simulink model "HR_Stateflow_Control"  (R2020b)
settings: Solver=VariableStepAuto  StartTime=0.0  StopTime=inf  MaxStep=1E-4  RelTol=1e-9
undefined symbols (not defined in the file): Dgain, g, Igain, initHeight, L1, L2, M, m1, m2, massTot, Pgain, physParam, tau1, tau2, th1o, th2o, yCMo
libraries: pid_lib x2, simulink x2
settings Model: Creator=Bradley Kwan  LastModifiedBy=Bradley Kwan
settings DebuggingCC: AlgebraicLoopMsg=none

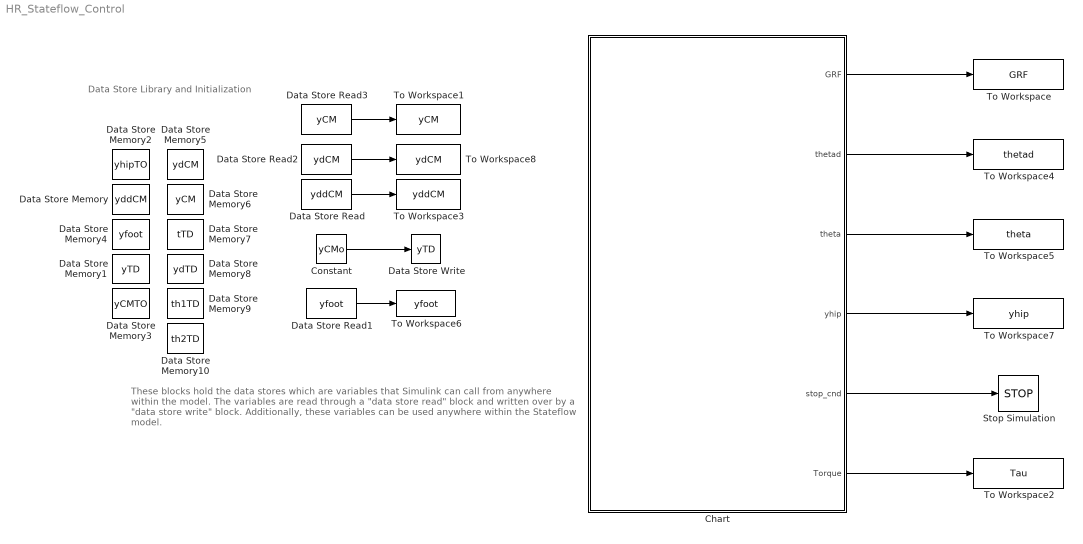
== system HR_Stateflow_Control ==
  note: These blocks hold the data stores which are variables that Simulink can call from anywhere within the model. The variables are read through a "data store read" block and written over by a "data store write" block. Additionally, these variables can be used anywhere within the Stateflow model.
  note: Data Store Library and Initialization
  Chart : Stateflow chart  TreatAsAtomicUnit=on
  Constant : Constant  Value=yCMo
  Data Store Memory : DataStoreMemory  DataStoreName=yddCM  ShowAdditionalParam=off  OutDataTypeStr=double
      settings: LockScale=on
  Data Store Memory1 : DataStoreMemory  DataStoreName=yTD  ShowAdditionalParam=off  OutDataTypeStr=double
      settings: LockScale=on
  Data Store Memory10 : DataStoreMemory  DataStoreName=th2TD  ShowAdditionalParam=off  OutDataTypeStr=double
      settings: LockScale=on
  Data Store Memory2 : DataStoreMemory  DataStoreName=yhipTO  ShowAdditionalParam=off  OutDataTypeStr=double
      settings: LockScale=on
  Data Store Memory3 : DataStoreMemory  DataStoreName=yCMTO  ShowAdditionalParam=off  OutDataTypeStr=double
      settings: LockScale=on
  Data Store Memory4 : DataStoreMemory  DataStoreName=yfoot  ShowAdditionalParam=off  OutDataTypeStr=double
      settings: LockScale=on
  Data Store Memory5 : DataStoreMemory  DataStoreName=ydCM  ShowAdditionalParam=off  OutDataTypeStr=double
      settings: LockScale=on
  Data Store Memory6 : DataStoreMemory  DataStoreName=yCM  ShowAdditionalParam=off  OutDataTypeStr=double
      settings: LockScale=on
  Data Store Memory7 : DataStoreMemory  DataStoreName=tTD  ShowAdditionalParam=off  OutDataTypeStr=double
      settings: LockScale=on
  Data Store Memory8 : DataStoreMemory  DataStoreName=ydTD  ShowAdditionalParam=off  OutDataTypeStr=double
      settings: LockScale=on
  Data Store Memory9 : DataStoreMemory  DataStoreName=th1TD  ShowAdditionalParam=off  OutDataTypeStr=double
      settings: LockScale=on
  Data Store Read : DataStoreRead  DataStoreName=yddCM
  Data Store Read1 : DataStoreRead  DataStoreName=yfoot
  Data Store Read2 : DataStoreRead  DataStoreName=ydCM
  Data Store Read3 : DataStoreRead  DataStoreName=yCM
  Data Store Write : DataStoreWrite  DataStoreName=yTD
  Stop Simulation : Stop
  To Workspace : ToWorkspace  VariableName=GRF  SampleTime=-1
  To Workspace1 : ToWorkspace  VariableName=yCM  SampleTime=-1
  To Workspace2 : ToWorkspace  VariableName=Tau  SampleTime=-1
  To Workspace3 : ToWorkspace  VariableName=yddCM  SampleTime=-1
  To Workspace4 : ToWorkspace  VariableName=thetad  SampleTime=-1
  To Workspace5 : ToWorkspace  VariableName=theta  SampleTime=-1
  To Workspace6 : ToWorkspace  VariableName=yfoot  SampleTime=-1
  To Workspace7 : ToWorkspace  VariableName=yhip  SampleTime=-1
  To Workspace8 : ToWorkspace  VariableName=ydCM  SampleTime=-1
  wires:
  Chart/1(GRF) -> To Workspace/1
  Chart/5(stop_cnd) -> Stop Simulation/1
  Data Store Read/1 -> To Workspace3/1
  Chart/2(thetad) -> To Workspace4/1
  Chart/3(theta) -> To Workspace5/1
  Constant/1 -> Data Store Write/1
  Chart/4(yhip) -> To Workspace7/1
  Data Store Read1/1 -> To Workspace6/1
  Data Store Read2/1 -> To Workspace8/1
  Data Store Read3/1 -> To Workspace1/1
  Chart/6(Torque) -> To Workspace2/1

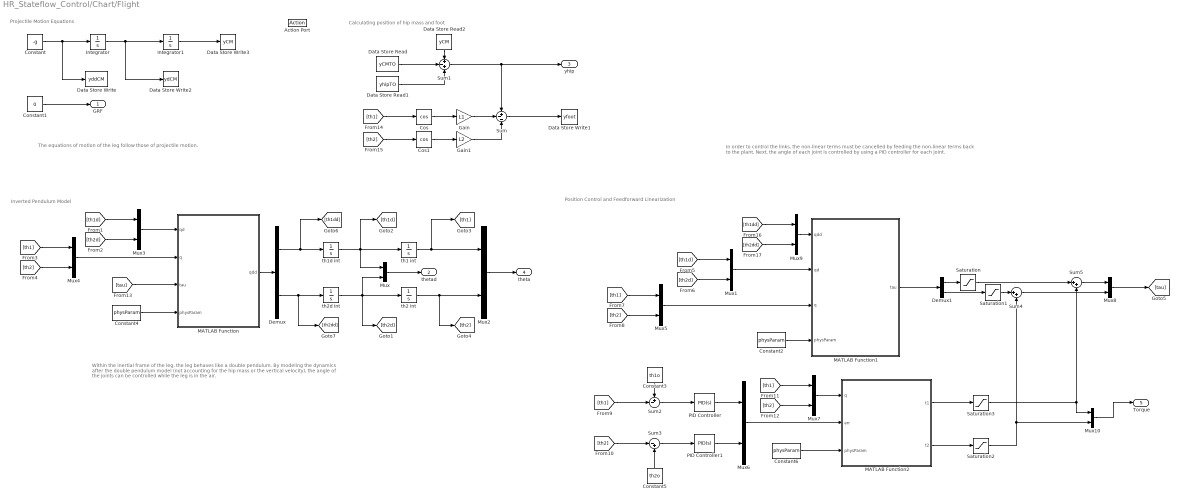
== system HR_Stateflow_Control/Chart/Flight ==
  note: The equations of motion of the leg follow those of projectile motion.
  note: In order to control the links, the non-linear terms must be cancelled by feeding the non-linear terms back to the plant. Next, the angle of each joint is controlled by using a PID controller for each joint.
  note: Within the inertial frame of the leg, the leg behaves like a double pendulum. By modeling the dynamics after the double pendulum model (not accounting for the hip mass or the vertical velocity), the angle of the joints can be controlled while the leg is in the air.
  note: Position Control and Feedforward Linearization
  note: Inverted Pendulum Model
  note: Calculating position of hip mass and foot
  note: Projectile Motion Equations
  Action Port : ActionPort
      settings: CopyFcn=Stateflow.SLINSF.SimulinkMan.removeBlockPreDeleteFcn  PreDeleteFcn=Stateflow.SLINSF.SimulinkMan.unsafePredeleteFcn
  Constant : Constant  Value=-g
  Constant1 : Constant  Value=0
  Constant2 : Constant  Value=physParam
  Constant3 : Constant  Value=th1o
  Constant4 : Constant  Value=physParam
  Constant5 : Constant  Value=th2o
  Constant6 : Constant  Value=physParam
  Cos : Trigonometry  Operator=cos
  Cos1 : Trigonometry  Operator=cos
  Data Store Read : DataStoreRead  DataStoreName=yCMTO
  Data Store Read1 : DataStoreRead  DataStoreName=yhipTO
  Data Store Read2 : DataStoreRead  DataStoreName=yCM
  Data Store Write : DataStoreWrite  DataStoreName=yddCM
  Data Store Write1 : DataStoreWrite  DataStoreName=yfoot
  Data Store Write2 : DataStoreWrite  DataStoreName=ydCM
  Data Store Write3 : DataStoreWrite  DataStoreName=yCM
  Demux : Demux  Outputs=2
  Demux1 : Demux  Outputs=2
  Gain : Gain  Gain=L1
  Gain1 : Gain  Gain=L2
  Integrator : Integrator  ContinuousStateAttributes='ydCM'
  Integrator1 : Integrator  InitialCondition=initHeight  ContinuousStateAttributes='yCM'
  MATLAB Function : MATLAB Function  TreatAsAtomicUnit=on
  MATLAB Function1 : MATLAB Function  TreatAsAtomicUnit=on
  MATLAB Function2 : MATLAB Function  TreatAsAtomicUnit=on
  Mux{,1..10} (11 alike) : Mux  Inputs=2
  PID Controller : pid_lib/PID Controller  Controller=PID  Form=Parallel  TimeDomain=Continuous-time  UseExternalTs=off  SampleTime=-1  IntegratorMethod=Forward Euler  FilterMethod=Forward Euler  ControllerParametersSource=internal  P=Pgain  I=Igain  D=Dgain  UseFilter=on  N=100  TunerSelectOption=Transfer Function Based (PID Tuner App)  InitialConditionSource=internal  InitialConditionForIntegrator=0  InitialConditionForFilter=0  DifferentiatorICPrevScaledInput=0  ExternalReset=none  TrackingMode=off  Kt=1  LimitOutput=off  SatLimitsSource=internal  UpperSaturationLimit=inf  LowerSaturationLimit=-inf  LinearizeAsGain=on  AntiWindupMode=none  Kb=1  POutMin=[]  POutMax=[]  IOutMin=[]  IOutMax=[]  DOutMin=[]  DOutMax=[]  NOutMin=[]  NOutMax=[]  SumOutMin=[]  SumOutMax=[]  SaturationOutMin=[]  SaturationOutMax=[]  PParamMin=[]  PParamMax=[]  IParamMin=[]  IParamMax=[]  DParamMin=[]  DParamMax=[]  NParamMin=[]  NParamMax=[]  KbParamMin=[]  KbParamMax=[]  KtParamMin=[]  KtParamMax=[]  KbOutMin=[]  KbOutMax=[]  KtOutMin=[]  KtOutMax=[]  IntegratorOutMin=[]  IntegratorOutMax=[]  FilterOutMin=[]  FilterOutMax=[]  SumI1OutMin=[]  SumI1OutMax=[]  SumI2OutMin=[]  SumI2OutMax=[]  SumI3OutMin=[]  SumI3OutMax=[]  SumI4OutMin=[]  SumI4OutMax=[]  SumDOutMin=[]  SumDOutMax=[]  DifferentiatorOutMin=[]  DifferentiatorOutMax=[]  FilterDiffOutCoefMin=[]  FilterDiffOutCoefMax=[]  ReciprocalOutMin=[]  ReciprocalOutMax=[]  SumDenOutMin=[]  SumDenOutMax=[]  SumNumOutMin=[]  SumNumOutMax=[]  DivideOutMin=[]  DivideOutMax=[]  UdiffTsProdOutMin=[]  UdiffTsProdOutMax=[]  NTsProdOutMin=[]  NTsProdOutMax=[]  UintegralTsProdOutMin=[]  UintegralTsProdOutMax=[]  UngainTsProdOutMin=[]  UngainTsProdOutMax=[]  IntegratorContinuousStateAttributes=''  IntegratorStateMustResolveToSignalObject=off  IntegratorRTWStateStorageClass=Auto  FilterContinuousStateAttributes=''  FilterStateMustResolveToSignalObject=off  FilterRTWStateStorageClass=Auto  ParallelPVariant=InternalParameters  IdealPVariant=Disabled  IVariant=InternalParameters  DVariant=InternalParameters  IntegratorVariant=Continuous  SatVariant=Disabled  AWVariant=Passthrough  PCopyVariant=Disabled  TRVariant=Disabled  FdbkBlocksVariant=Forward  IdealPFdbkVariant=Disabled  SatFdbkVariant=Disabled  DerivativeFilterVariant=ContFilter  NVariant=InternalParameters  NCopyVariant=Disabled  FilterICVariant=InternalICsFilter  IntegratorICVariant=InternalICs  ExternalResetVariant=Disabled  TRSumVariant=Passthrough  SumFdbkVariant=Disabled  SumVariant=Sum_PID  TsampFilterVariant=InternalTs  TsampNgainVariant=Passthrough  TsampIntegralVariant=Passthrough  ExternalSaturationOutDataTypeStr=Inherit: Same as second input
  PID Controller1 : pid_lib/PID Controller  Controller=PID  Form=Parallel  TimeDomain=Continuous-time  UseExternalTs=off  SampleTime=-1  IntegratorMethod=Forward Euler  FilterMethod=Forward Euler  ControllerParametersSource=internal  P=Pgain  I=Igain  D=Dgain  UseFilter=on  N=100  TunerSelectOption=Transfer Function Based (PID Tuner App)  InitialConditionSource=internal  InitialConditionForIntegrator=0  InitialConditionForFilter=0  DifferentiatorICPrevScaledInput=0  ExternalReset=none  TrackingMode=off  Kt=1  LimitOutput=off  SatLimitsSource=internal  UpperSaturationLimit=inf  LowerSaturationLimit=-inf  LinearizeAsGain=on  AntiWindupMode=none  Kb=1  POutMin=[]  POutMax=[]  IOutMin=[]  IOutMax=[]  DOutMin=[]  DOutMax=[]  NOutMin=[]  NOutMax=[]  SumOutMin=[]  SumOutMax=[]  SaturationOutMin=[]  SaturationOutMax=[]  PParamMin=[]  PParamMax=[]  IParamMin=[]  IParamMax=[]  DParamMin=[]  DParamMax=[]  NParamMin=[]  NParamMax=[]  KbParamMin=[]  KbParamMax=[]  KtParamMin=[]  KtParamMax=[]  KbOutMin=[]  KbOutMax=[]  KtOutMin=[]  KtOutMax=[]  IntegratorOutMin=[]  IntegratorOutMax=[]  FilterOutMin=[]  FilterOutMax=[]  SumI1OutMin=[]  SumI1OutMax=[]  SumI2OutMin=[]  SumI2OutMax=[]  SumI3OutMin=[]  SumI3OutMax=[]  SumI4OutMin=[]  SumI4OutMax=[]  SumDOutMin=[]  SumDOutMax=[]  DifferentiatorOutMin=[]  DifferentiatorOutMax=[]  FilterDiffOutCoefMin=[]  FilterDiffOutCoefMax=[]  ReciprocalOutMin=[]  ReciprocalOutMax=[]  SumDenOutMin=[]  SumDenOutMax=[]  SumNumOutMin=[]  SumNumOutMax=[]  DivideOutMin=[]  DivideOutMax=[]  UdiffTsProdOutMin=[]  UdiffTsProdOutMax=[]  NTsProdOutMin=[]  NTsProdOutMax=[]  UintegralTsProdOutMin=[]  UintegralTsProdOutMax=[]  UngainTsProdOutMin=[]  UngainTsProdOutMax=[]  IntegratorContinuousStateAttributes=''  IntegratorStateMustResolveToSignalObject=off  IntegratorRTWStateStorageClass=Auto  FilterContinuousStateAttributes=''  FilterStateMustResolveToSignalObject=off  FilterRTWStateStorageClass=Auto  ParallelPVariant=InternalParameters  IdealPVariant=Disabled  IVariant=InternalParameters  DVariant=InternalParameters  IntegratorVariant=Continuous  SatVariant=Disabled  AWVariant=Passthrough  PCopyVariant=Disabled  TRVariant=Disabled  FdbkBlocksVariant=Forward  IdealPFdbkVariant=Disabled  SatFdbkVariant=Disabled  DerivativeFilterVariant=ContFilter  NVariant=InternalParameters  NCopyVariant=Disabled  FilterICVariant=InternalICsFilter  IntegratorICVariant=InternalICs  ExternalResetVariant=Disabled  TRSumVariant=Passthrough  SumFdbkVariant=Disabled  SumVariant=Sum_PID  TsampFilterVariant=InternalTs  TsampNgainVariant=Passthrough  TsampIntegralVariant=Passthrough  ExternalSaturationOutDataTypeStr=Inherit: Same as second input
  Saturation : Saturate  UpperLimit=8  LowerLimit=-8
  Saturation1 : Saturate  UpperLimit=8  LowerLimit=-8
  Saturation2 : Saturate  UpperLimit=5  LowerLimit=-5
  Saturation3 : Saturate  UpperLimit=5  LowerLimit=-5
  Sum : Sum  Inputs=+--
  Sum1 : Sum  Inputs=+-+
  Sum2 : Sum  Inputs=+-|
  Sum3 : Sum  Inputs=|-+
  Sum4 : Sum  Inputs=|++
  Sum5 : Sum  Inputs=|++
  th1 int : Integrator  InitialCondition=th1o  ContinuousStateAttributes='th1'
  th1d int : Integrator  ContinuousStateAttributes='th1d'
  th2 int : Integrator  InitialCondition=th2o  ContinuousStateAttributes='th2'
  th2d int : Integrator  ContinuousStateAttributes='th2d'
  GRF : Outport
  thetad : Outport  Port=2
  yhip : Outport  Port=3
  theta : Outport  Port=4
  Torque : Outport  Port=5
  wires:
  Constant1/1 -> GRF/1
  Constant/1 -> Data Store Write/1, Integrator/1
  Integrator/1 -> Data Store Write2/1, Integrator1/1
  Integrator1/1 -> Data Store Write3/1
  Cos/1 -> Gain/1
  Cos1/1 -> Gain1/1
  Gain/1 -> Sum/2
  Gain1/1 -> Sum/3
  Sum/1 -> Data Store Write1/1
  Data Store Read/1 -> Sum1/2
  Data Store Read2/1 -> Sum1/1
  Data Store Read1/1 -> Sum1/3
  Sum1/1 -> Sum/1, yhip/1
  MATLAB Function/1(qdd) -> Demux/1
  th1d int/1 -> Mux/1, th1 int/1, [th1d]
  th2d int/1 -> Mux/2, [th2d], th2 int/1
  th1 int/1 -> [th1], Mux2/1
  th2 int/1 -> [th2], Mux2/2
  Constant4/1 -> MATLAB Function/4(physParam)
  [th1d] -> Mux3/1
  [th2d] -> Mux3/2
  Mux3/1 -> MATLAB Function/1(qd)
  [th2] -> Mux4/2
  [th1] -> Mux4/1
  Mux4/1 -> MATLAB Function/2(q)
  Constant2/1 -> MATLAB Function1/4(physParam)
  Mux5/1 -> MATLAB Function1/3(q)
  [th1] -> Mux5/1
  [th2] -> Mux5/2
  Mux1/1 -> MATLAB Function1/2(qd)
  [th2d] -> Mux1/2
  [th1d] -> Mux1/1
  MATLAB Function1/1(tau) -> Demux1/1
  [th2] -> Sum3/1
  [th1] -> Sum2/2
  Constant3/1 -> Sum2/1
  Constant5/1 -> Sum3/2
  Sum2/1 -> PID Controller/1
  Sum3/1 -> PID Controller1/1
  PID Controller/1 -> Mux6/1
  PID Controller1/1 -> Mux6/2
  Mux6/1 -> MATLAB Function2/2(err)
  [th2] -> Mux7/2
  [th1] -> Mux7/1
  Mux7/1 -> MATLAB Function2/1(q)
  Constant6/1 -> MATLAB Function2/3(physParam)
  Mux2/1 -> theta/1
  MATLAB Function2/1(t1) -> Saturation3/1
  Sum5/1 -> Mux8/1
  Sum4/1 -> Mux8/2
  Mux8/1 -> [tau]
  [tau] -> MATLAB Function/3(tau)
  Demux/1 -> [th1dd], th1d int/1
  Demux/2 -> [th2dd], th2d int/1
  [th1] -> Cos/1
  [th2] -> Cos1/1
  Mux/1 -> thetad/1
  Demux1/1 -> Saturation/1
  Saturation/1 -> Sum5/1
  Demux1/2 -> Saturation1/1
  Saturation1/1 -> Sum4/1
  [th1dd] -> Mux9/1
  [th2dd] -> Mux9/2
  Mux9/1 -> MATLAB Function1/1(qdd)
  Mux10/1 -> Torque/1
  MATLAB Function2/2(t2) -> Saturation2/1
  Saturation3/1 -> Sum5/2, Mux10/1
  Saturation2/1 -> Sum4/2, Mux10/2

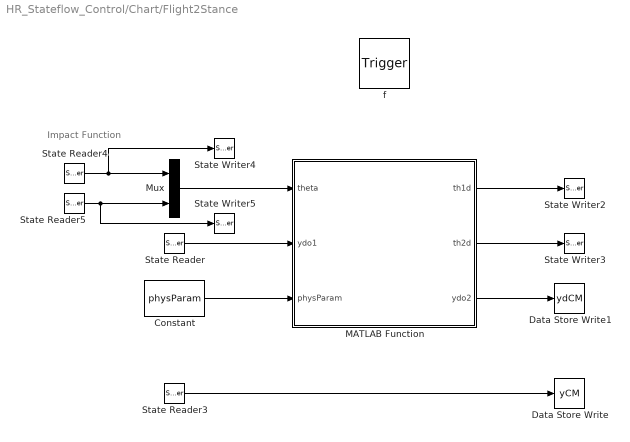
== system HR_Stateflow_Control/Chart/Flight2Stance ==
  note: Impact Function
  f : TriggerPort  TriggerType=function-call  VariantControl=(inherit)
      settings: CopyFcn=Stateflow.SLINSF.SimulinkMan.removeBlockPreDeleteFcn  PreDeleteFcn=Stateflow.SLINSF.SimulinkMan.unsafePredeleteFcn
  Constant : Constant  Value=physParam
  Data Store Write : DataStoreWrite  DataStoreName=yCM
  Data Store Write1 : DataStoreWrite  DataStoreName=ydCM
  MATLAB Function : MATLAB Function  TreatAsAtomicUnit=on
  Mux : Mux  Inputs=2
  State Reader : StateReader  StateOwnerBlock=../../Flight/Integrator  StateName=ydCM
  State Reader3 : StateReader  StateOwnerBlock=../../Flight/Integrator1  StateName=yCM
  State Reader4 : StateReader  StateOwnerBlock=../../Flight/th1 int  StateName=th1
  State Reader5 : StateReader  StateOwnerBlock=../../Flight/th2 int  StateName=th2
  State Writer2 : StateWriter  StateOwnerBlock=../../Stance/th1d int.  StateName=th1d
  State Writer3 : StateWriter  StateOwnerBlock=../../Stance/th2d int.  StateName=th2d
  State Writer4 : StateWriter  StateOwnerBlock=../../Stance/th1 int.  StateName=th1
  State Writer5 : StateWriter  StateOwnerBlock=../../Stance/th2 int.  StateName=th2
  wires:
  State Reader/1 -> MATLAB Function/2(ydo1)
  State Reader4/1 -> Mux/1, State Writer4/1
  Mux/1 -> MATLAB Function/1(theta)
  Constant/1 -> MATLAB Function/3(physParam)
  MATLAB Function/3(ydo2) -> Data Store Write1/1
  State Reader3/1 -> Data Store Write/1
  MATLAB Function/1(th1d) -> State Writer2/1
  MATLAB Function/2(th2d) -> State Writer3/1
  State Reader5/1 -> Mux/2, State Writer5/1

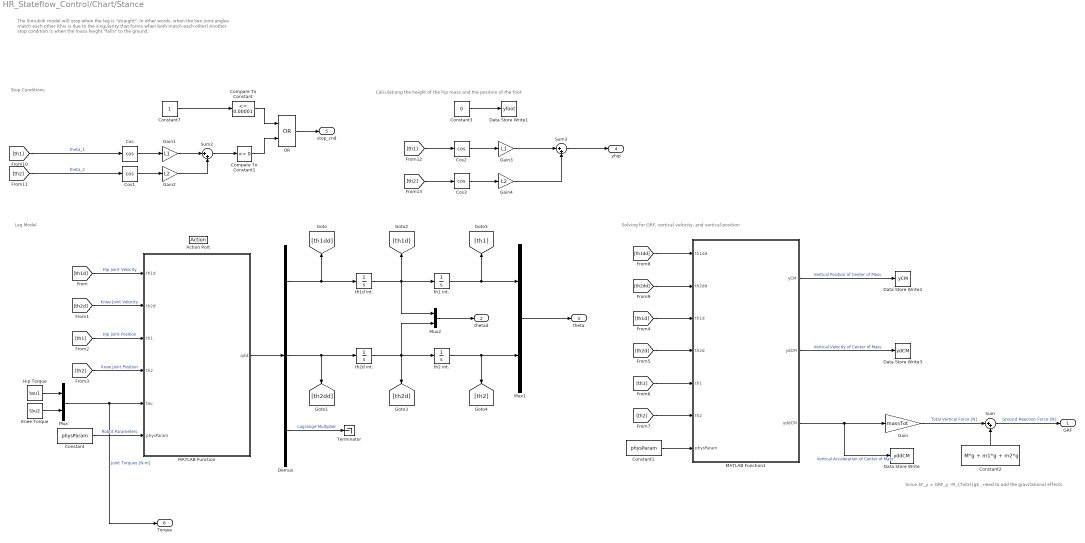
== system HR_Stateflow_Control/Chart/Stance ==
  note: Calculatiung the height of the hip mass and the position of the foot
  note: Solving for GRF, vertical velocity, and vertical position
  note: Leg Model
  note: Since $F_y = GRF_y -M_{Total}g$ , need to add the gravitational effects
  note: Stop Conditions
  note: The Simulink model will stop when the leg is "straight". In other words, when the two joint angles match each other (this is due to the singularity that forms when both match each other)
      |
      | Another stop condition is when the mass height "falls" to the ground.
  Action Port : ActionPort
      settings: CopyFcn=Stateflow.SLINSF.SimulinkMan.removeBlockPreDeleteFcn  PreDeleteFcn=Stateflow.SLINSF.SimulinkMan.unsafePredeleteFcn
  Compare To Constant : simulink/Logic and Bit Operations/Compare To Constant  relop=<=  const=0.00001  OutDataTypeStr=boolean
  Compare To Constant1 : simulink/Logic and Bit Operations/Compare To Constant  relop=<=  const=0  OutDataTypeStr=boolean
  Constant : Constant  Value=physParam
  Constant1 : Constant  Value=physParam
  Constant2 : Constant  Value=M*g + m1*g + m2*g
  Constant3 : Constant  Value=0
  Constant7 : Constant
  Cos{,1..3} (4 alike) : Trigonometry  Operator=cos
  Data Store Write : DataStoreWrite  DataStoreName=yddCM
  Data Store Write1 : DataStoreWrite  DataStoreName=yfoot
  Data Store Write2 : DataStoreWrite  DataStoreName=yCM
  Data Store Write3 : DataStoreWrite  DataStoreName=ydCM
  Demux : Demux  Outputs=3
  Gain : Gain  Gain=massTot
  Gain1 : Gain  Gain=L1
  Gain2 : Gain  Gain=L2
  Gain3 : Gain  Gain=L1
  Gain4 : Gain  Gain=L2
  Hip Torque : Constant  Value=tau1
  Knee Torque : Constant  Value=tau2
  MATLAB Function : MATLAB Function  TreatAsAtomicUnit=on
  MATLAB Function1 : MATLAB Function  TreatAsAtomicUnit=on
  Mux : Mux  Inputs=2
  Mux1 : Mux  Inputs=2
  Mux2 : Mux  Inputs=2
  OR : Logic  Operator=OR  IconShape=distinctive  AllPortsSameDT=off  OutDataTypeStr=boolean
  Sum : Sum  Inputs=|++
  Sum2 : Sum  Inputs=|++
  Sum3 : Sum  Inputs=|++
  Terminator : Terminator
  th1 int. : Integrator  InitialCondition=th1o  ContinuousStateAttributes='th1'
  th1d int. : Integrator  ContinuousStateAttributes='th1d'
  th2 int. : Integrator  InitialCondition=th2o  ContinuousStateAttributes='th2'
  th2d int. : Integrator  ContinuousStateAttributes='th2d'
  GRF : Outport
  thetad : Outport  Port=2
  theta : Outport  Port=3
  yhip : Outport  Port=4
  stop_cnd : Outport  Port=5
  Torque : Outport  Port=6
  wires:
  Knee Torque/1 -> Mux/2
  Hip Torque/1 -> Mux/1
  Mux/1 -> Torque/1, MATLAB Function/5(tau)  "Joint Torques [N-m]"
  Constant/1 -> MATLAB Function/6(physParam)  "Robot Parameters"
  [th1d] -> MATLAB Function/1(th1d)  "Hip Joint Velocity"
  [th2d] -> MATLAB Function/2(th2d)  "Knee Joint Velocity"
  [th1] -> MATLAB Function/3(th1)  "Hip Joint Position"
  [th2] -> MATLAB Function/4(th2)  "Knee Joint Position"
  MATLAB Function/1(qdd) -> Demux/1
  Demux/1 -> [th1dd], th1d int./1
  Demux/2 -> [th2dd], th2d int./1
  th1d int./1 -> Mux2/1, th1 int./1, [th1d]
  th2d int./1 -> Mux2/2, [th2d], th2 int./1
  Mux1/1 -> theta/1
  th1 int./1 -> [th1], Mux1/1
  th2 int./1 -> [th2], Mux1/2
  Demux/3 -> Terminator/1  "Lagrange Multiplier"
  Mux2/1 -> thetad/1
  Constant1/1 -> MATLAB Function1/7(physParam)
  [th2] -> MATLAB Function1/6(th2)
  [th1] -> MATLAB Function1/5(th1)
  [th2d] -> MATLAB Function1/4(th2d)
  [th1d] -> MATLAB Function1/3(th1d)
  [th2dd] -> MATLAB Function1/2(th2dd)
  [th1dd] -> MATLAB Function1/1(th1dd)
  MATLAB Function1/3(yddCM) -> Data Store Write/1, Gain/1  "Vertical Acceleration of Center of Mass"
  Gain/1 -> Sum/1  "Total Vertical Force [N]"
  Constant2/1 -> Sum/2
  Gain2/1 -> Sum2/2
  OR/1 -> stop_cnd/1
  Compare To Constant/1 -> OR/1
  Cos1/1 -> Gain2/1
  [th1] -> Cos/1  "theta_1"
  [th2] -> Cos1/1  "theta_2"
  Sum2/1 -> Compare To Constant1/1
  Cos/1 -> Gain1/1
  Compare To Constant1/1 -> OR/2
  Gain1/1 -> Sum2/1
  Sum/1 -> GRF/1  "Ground Reaction Force [N]"
  Constant3/1 -> Data Store Write1/1
  [th1] -> Cos2/1
  [th2] -> Cos3/1
  Cos2/1 -> Gain3/1
  Cos3/1 -> Gain4/1
  Gain3/1 -> Sum3/1
  Gain4/1 -> Sum3/2
  Sum3/1 -> yhip/1
  MATLAB Function1/1(yCM) -> Data Store Write2/1  "Vertical Position of Center of Mass"
  MATLAB Function1/2(ydCM) -> Data Store Write3/1  "Vertical Velocity of Center of Mass"
  Constant7/1 -> Compare To Constant/1

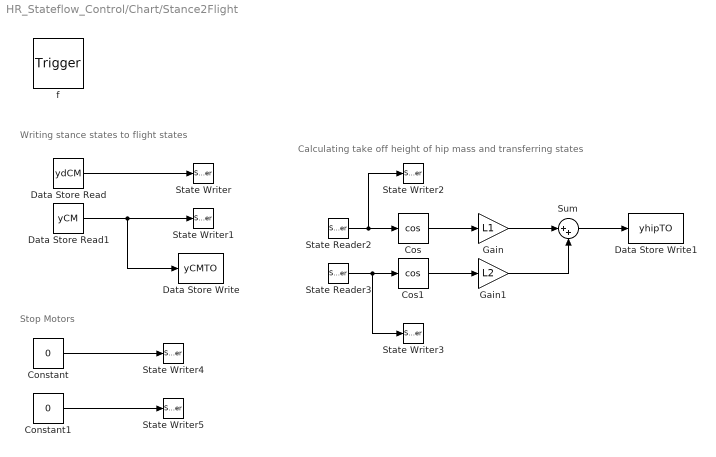
== system HR_Stateflow_Control/Chart/Stance2Flight ==
  note: Calculating take off height of hip mass and transferring states
  note: Writing stance states to flight states
  note: Stop Motors
  f : TriggerPort  TriggerType=function-call  VariantControl=(inherit)
      settings: CopyFcn=Stateflow.SLINSF.SimulinkMan.removeBlockPreDeleteFcn  PreDeleteFcn=Stateflow.SLINSF.SimulinkMan.unsafePredeleteFcn
  Constant : Constant  Value=0
  Constant1 : Constant  Value=0
  Cos : Trigonometry  Operator=cos
  Cos1 : Trigonometry  Operator=cos
  Data Store Read : DataStoreRead  DataStoreName=ydCM
  Data Store Read1 : DataStoreRead  DataStoreName=yCM
  Data Store Write : DataStoreWrite  DataStoreName=yCMTO
  Data Store Write1 : DataStoreWrite  DataStoreName=yhipTO
  Gain : Gain  Gain=L1
  Gain1 : Gain  Gain=L2
  State Reader2 : StateReader  StateOwnerBlock=../../Stance/th1 int.  StateName=th1
  State Reader3 : StateReader  StateOwnerBlock=../../Stance/th2 int.  StateName=th2
  State Writer : StateWriter  StateOwnerBlock=../../Flight/Integrator  StateName=ydCM
  State Writer1 : StateWriter  StateOwnerBlock=../../Flight/Integrator1  StateName=yCM
  State Writer2 : StateWriter  StateOwnerBlock=../../Flight/th1 int  StateName=th1
  State Writer3 : StateWriter  StateOwnerBlock=../../Flight/th2 int  StateName=th2
  State Writer4 : StateWriter  StateOwnerBlock=../../Flight/th1d int  StateName=th1d
  State Writer5 : StateWriter  StateOwnerBlock=../../Flight/th2d int  StateName=th2d
  Sum : Sum  Inputs=|++
  wires:
  Data Store Read/1 -> State Writer/1
  Gain1/1 -> Sum/2
  Gain/1 -> Sum/1
  Cos1/1 -> Gain1/1
  State Reader2/1 -> State Writer2/1, Cos/1
  Sum/1 -> Data Store Write1/1
  Cos/1 -> Gain/1
  Data Store Read1/1 -> Data Store Write/1, State Writer1/1
  State Reader3/1 -> State Writer3/1, Cos1/1
  Constant/1 -> State Writer4/1
  Constant1/1 -> State Writer5/1

== matlab function HR_Stateflow_Control/Chart/Flight2Stance/MATLAB Function ==
  data: theta input; th1d output; ydo1 input; physParam input; th2d output; ydo2 output
function [th1d, th2d, ydo2] = flightimpact(theta,ydo1,physParam)

    % Assigning physical parameters to variables
    L1 = physParam(1);
    L2 = physParam(2);
    m1 = physParam(3);
    m2 = physParam(4);
    M  = physParam(5);
    th1 = theta(1);
    th2 = theta(2);
    
    % Vectorizing y velocity
    vleg = [0 ydo1 0];

    % Mass moment of inertia of respective links
    I1 = 1/12*m1*L1^2;
    I2 = 1/12*m2*L2^2;

    % First the distance vectors need to be determined for the conservation of
    % momentum equation [Origin placed on ground directly below hip mass.

    % Distance from origin to thigh link
    rog1 = [L1/2*sin(th1) L2*cos(th2)+L1/2*cos(th1) 0];
    % Distance from origin to shank link
    rog2 = [L1*sin(th1)+L2/2*sin(th2) L2/2*cos(th2) 0];
    % Distance from origin to hip mass
    roM  = [0 L1*cos(th1)+L2*cos(th2) 0];

    % Performing cross product
    Lm1 = cross(rog1,m1*vleg);
    Lm2 = cross(rog2,m2*vleg);
    LM  = cross(roM, M*vleg);
    
    flightL = Lm1+Lm2+LM;
    A =zeros(6,7);
    % Setting up conservation of angular momentum equation
    A(1,:) = [I1 I2  -rog1(2)*m1 rog1(1)*m1 -rog2(2)*m2 rog2(1)*m2 flightL(3)];
    % Non-holonomic constraint
    A(2,:) = [L1*cos(th1) L2*cos(th2) 0 0 0 0 0];
    % Horizontal velocity of thigh link
    A(3,:) = [L1/2*cos(th1) 0 -1 0 0 0 0];
    % Vertical velocity of thigh link
    A(4,:) = [L1/2*sin(th1) L2*sin(th2) 0 1 0 0 0];
    % Horizontal velocity of thigh link
    A(5,:) = [L1*cos(th1) L2/2*cos(th2) 0 0 -1 0 0];
    % Vertical velocity of thigh link
    A(6,:) = [0 L2/2*sin(th2) 0 0 0 1 0];

    mysoln = linsolve(A(1:6,1:6),A(:,7));
    th1d  = mysoln(1);
    th2d  = mysoln(2);
    % Solving for new vertical velocity of center of mass [m/s]
    ydM = -(L1*sin(th1).*th1d+L2*sin(th2).*th2d);
    ydm1 = mysoln(4);
    ydm2 = mysoln(6);
    ydo2 = 1/(m1+m2+M)*(m1*ydm1+m2*ydm2+M*ydM);
end

== matlab function HR_Stateflow_Control/Chart/Flight/MATLAB Function ==
  data: qd input; qdd output; q input; tau input; physParam input
function qdd = Leg_Dynamics(qd, q, tau, physParam)
g = 9.81;    % gravitational acceleration [m/s^2]

th1  = q(1);
th2  = q(2);
th1d = qd(1);
th2d = qd(2);
tau1 = tau(1);
tau2 = tau(2);

L1 = physParam(1);
L2 = physParam(2);
m1 = physParam(3);
m2 = physParam(4);
M  = physParam(5);

I1 = 1/12*m1*L1^2;
I2 = 1/12*m2*L2^2;

% Inertia matrix
B = [(L1^2*(m1+4*m2))/4,  L1*L2*m2*cos(th1-th2)/2;
    L1*L2*m2*cos(th1-th2)/2, L2^2*m2/4];

% Centrifugal effects
C = [L1*L2*m2*th2d*sin(th1-th2)/2, -L1*L2*m2*th2d*sin(th1-th2)/2
     L1*L2*m2*sin(th1-th2)*th1d/2, -L1*L2*m2*th1d*sin(th1-th2)/2];
% Components due to gravitational effects
D = [-L1*g*sin(th1)*(m1/2+m2); -L2*g*m2*sin(th2)/2];


qdd = inv(B)*[tau1;tau2] - inv(B)*C*[qd] - inv(B)*D;

== matlab function HR_Stateflow_Control/Chart/Flight/MATLAB Function1 ==
  data: qdd input; qd input; tau output; q input; physParam input
function tau = linearizeTau(qdd, qd, q, physParam)

g = 9.81;

% States of manipulator
th1  = q(1);
th2  = q(2);
th1d = qd(1);
th2d = qd(2);

% Define physical parameters of manipulator
L1 = physParam(1);
L2 = physParam(2);
m1 = physParam(3);
m2 = physParam(4);
M  = physParam(5);

% Non-linear terms from generalized inertia matrix
B = [0,  L1*L2*m2*cos(th1-th2)/2;
     L1*L2*m2*cos(th1-th2)/2, 0];

% Centrifugal effects
C = [L1*L2*m2*th2d*sin(th1-th2)/2, -L1*L2*m2*th2d*sin(th1-th2)/2
     L1*L2*m2*sin(th1-th2)*th1d/2, -L1*L2*m2*th1d*sin(th1-th2)/2];
% Components due to gravitational effects
D = [-L1*g*sin(th1)*(m1/2+m2); -L2*g*m2*sin(th2)/2];

% Calculating torque (without the PID controller terms)
tau = B*qdd + C*qd + D;

== matlab function HR_Stateflow_Control/Chart/Flight/MATLAB Function2 ==
  data: q input; err input; t1 output; physParam input; t2 output
function [t1, t2] = Leg_Dynamics(q, err, physParam)
th1  = q(1);
th2  = q(2);

L1 = physParam(1);
L2 = physParam(2);
m1 = physParam(3);
m2 = physParam(4);
M  = physParam(5);

I1 = 1/12*m1*L1^2;
I2 = 1/12*m2*L2^2;

% Inertia matrix
B = [(L1^2*(m1+4*m2))/4, 0;
      0, L2^2*m2/4];
 
mytau = B*err;
t1 = mytau(1);
t2 = mytau(2);

== matlab function HR_Stateflow_Control/Chart/Stance/MATLAB Function1 ==
  data: yCM output; ydCM output; th1dd input; yddCM output; th2dd input; th1d input; th2d input; th1 input; th2 input; physParam input
function [yCM, ydCM, yddCM]   = vertAccel(th1dd, th2dd, th1d, th2d, th1, th2,physParam)

% Define physical parameters of leg

L1 = physParam(1);
L2 = physParam(2);
m1 = physParam(3);
m2 = physParam(4);
M  = physParam(5);

yM  = L1*cos(th1) + L2*cos(th2);
ym1 = L1/2*cos(th1)+L2*cos(th2);
ym2 = L2/2*cos(th2);
yCM = 1/(m1+m2+M)*(M*yM+m1*ym1+m2*ym2);

ydM  = -(L1*sin(th1)*th1d + L2*sin(th2)*th2d);
ydm1 = -(L1/2*sin(th1)*th1d + L2*sin(th2)*th2d);
ydm2 = -L2/2*sin(th2)*th2d;
ydCM = 1/(m1+m2+M)*(M*ydM+m1*ydm1+m2*ydm2);

yddM = -L1*(cos(th1)*th1d^2+sin(th1)*th1dd)-(L2*(cos(th2)*th2d^2+sin(th2)*th2dd));
yddm1 = -L1/2*(cos(th1)*th1d^2+sin(th1)*th1dd)-L2*(cos(th2)*th2d^2+sin(th2)*th2dd);
yddm2 = -L2/2*(cos(th2)*th2d^2+sin(th2)*th2dd);
yddCM = 1/(m1+m2+M)*(M*yddM+m1*yddm1+m2*yddm2);

== matlab function HR_Stateflow_Control/Chart/Stance/MATLAB Function ==
  data: th1d input; qdd output; th2d input; th1 input; th2 input; tau input; physParam input
function qdd = Leg_Dynamics(th1d,th2d, th1, th2, tau, physParam)
g = 9.81;    % gravitational acceleration [m/s^2]
tau1 = tau(1);
tau2 = tau(2);
q = [th1 th2]';
qd = [th1d th2d]';

L1 = physParam(1);
L2 = physParam(2);
m1 = physParam(3);
m2 = physParam(4);
M  = physParam(5);

I1 = 1/12*m1*L1^2;
I2 = 1/12*m2*L2^2;

% Inertia matrix
B = [L1^2*(1/4*m1+I1+m2*cos(th1)^2+M*sin(th1)^2), L1*L2*((M+m1/2)*sin(th1)*sin(th2)+m2/2*cos(th1)*cos(th2)), -L1*cos(th1);
     L1*L2*((M+m1/2)*sin(th1)*sin(th2)+m2/2*cos(th1)*cos(th2)), L2^2*((M+m1)*sin(th2)^2+I2+1/4*m2), -L2*cos(th2);
     -L1*cos(th1), -L2*cos(th2), 0];

% Centrifugal effects
C = [(M-m2)*L1^2*cos(th1)*sin(th1)*th1d, L1*L2*th2d*(-m2/2*cos(th1)*sin(th2)+(M+m1/2)*cos(th2)*sin(th1)), 0;
     L1*L2*th1d*((M+m1/2)*cos(th1)*sin(th2)-m2*cos(th2)*sin(th1)), L2^2*th2d*(M+m1)*cos(th2)*sin(th2),0;
     L1*sin(th1)*th1d, L2*sin(th2)*th2d, 0];    

% Components due to gravitational effects
D = [-L1/2*g*sin(th1)*(2*M+m1); -L2*g*sin(th2)*(M+m1+m2/2); 0];


qdd = inv(B)*[tau1;tau2;0] - inv(B)*C*[qd;0] - inv(B)*D;

== stateflow chart HR_Stateflow_Control/Chart ==
  note: The Flight2Stance function accounts for the impact of the leg by taking the current position of the leg and vertical velocity of each component. This assigns a new vertical velocity to the center of mass and finds the appropriate link velocities. Additionally it writes the states from the flight state over to the corresponding states within the stance state.
  note: The Stance2Flight function saves the position of the center of mass and writes the states of the stance state to the corresponding states within the flight state.
  state Stance
  state Stance2Flight [function]
  state Flight2Stance [function]
  state Flight
  state Stop
    entry:
    stop_cnd = true;
  Stance -> Flight : [ydCM > 0  && yddCM < -9.81]{Stance2Flight;}
  Flight -> Stance [order 2] : [Flight.ydCM < 0 && yfoot <= 0]{Flight2Stance; hopCount = hopCount+1;}
  (default) -> Flight : {hopCount = 0; tTD = 0; ydTD = 0;}
  Flight -> Stop [order 1] : [hopCount == 100]
  data: sf_internal_action_state_placeholder_data local double size=1 =0; sf_internal_action_state_placeholder_data local double size=1 =0; ydCM local; GRF output; yddCM data_store_memory; thetad output; theta output; yhip output; stop_cnd output; yfoot data_store_memory; hopCount local; ydCM data_store_memory; tTD data_store_memory; ydTD data_store_memory; Torque output
